simulink model "ardrone_alphaepsilon"  (R2023b)
settings: configuration reference "AR_Drone_ConfigSet" (kept outside this file)
undefined symbols (not defined in the file or in its folder): accelerometerXyzGains, accelerometerXyzOffsets, DiscIntNeverNeededParam, gyroXyzOffsets, Mag_Calib_Gain_Vector, Mag_Calib_Offset_Vector
libraries: simulink x4, AR_Drone_Sensors x2, AR_Drone_Actuators x2, vrlib x2
settings Model: DataDictionary=ArDroneDataDictionary.sldd  EnableAccessToBaseWorkspace=off  SimulationMode=external  ExtModeTrigDuration=48000  Creator=nraman  LastModifiedBy=sonso
settings ConfigSetRef: SourceName=AR_Drone_ConfigSet

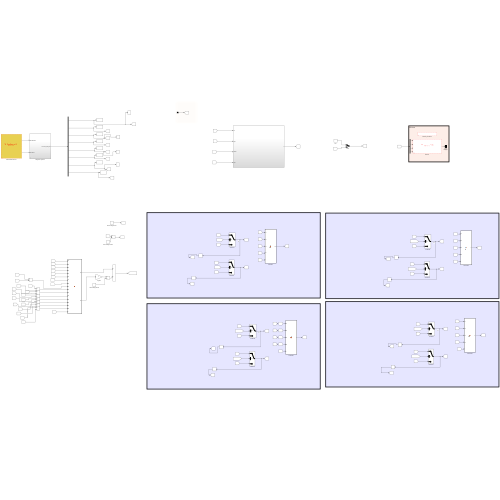
[thumbnail: Simulink's stored preview of the top-level diagram]
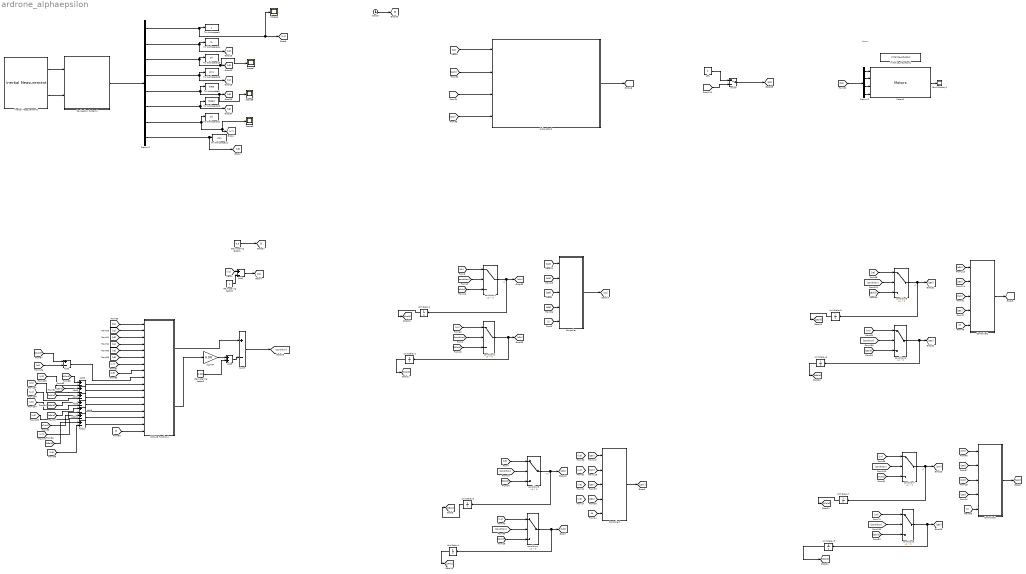
== system ardrone_alphaepsilon ==
  note: Motors
  note: x1
  note: x1
  note: x1
  note: x1
  Add{1..3,6..11} (9 alike) : Sum  Inputs=+-
  Add5 : Sum
  Clock5 : Clock
  Controller : MATLAB Function  TreatAsAtomicUnit=on
  Controller1 : MATLAB Function  TreatAsAtomicUnit=on
  Controller2 : MATLAB Function  TreatAsAtomicUnit=on
  Controller3 : MATLAB Function  TreatAsAtomicUnit=on
  Demux1 : Demux  Outputs=8
  Demux2 : Demux
  Fault Display1 : Display
  Gain-scaling factor1 : Constant  Value=0.5
  Gain-scaling factor2 : Constant
  Gain-scaling factor6 : Constant  Value=0.001
  Inertial Measurement1 : AR_Drone_Sensors/Inertial Measurement  Ts=1/400
  Initialize_Actuators1 : AR_Drone_Actuators/Initialize_Actuators  ShowSpec=on
  MATLAB Function4 : MATLAB Function  TreatAsAtomicUnit=on
  Motors1 : AR_Drone_Actuators/Motors
  Navigation System1 : Subsystem  AncestorBlock=AR_Drone_Positioning/Navigation System
  Scope{6..9} (4 alike) : Scope
  Subsystem2 : Subsystem
  Sum5 : Sum  Inputs=+-
  To Workspace10 : ToWorkspace  VariableName=theta1  SampleTime=-1
  To Workspace11 : ToWorkspace  VariableName=psi  SampleTime=-1
  To Workspace12 : ToWorkspace  VariableName=psi1  SampleTime=-1
  To Workspace14 : ToWorkspace  VariableName=z1  SampleTime=-1
  To Workspace16 : ToWorkspace  VariableName=phi  SampleTime=-1
  To Workspace18 : ToWorkspace  VariableName=phi1  SampleTime=-1
  To Workspace8 : ToWorkspace  VariableName=theta  SampleTime=-1
  To Workspace9 : ToWorkspace  VariableName=z  SampleTime=-1
  Unit Delay{1..8} (8 alike) : UnitDelay  SampleTime=-1  HasFrameUpgradeWarning=on
  condition{1..8} (8 alike) : Switch  Criteria=u2 > Threshold  SaturateOnIntegerOverflow=off  InputSameDT=off
  off1 : Constant  Value=0
  on/off : ManualSwitch
  sigma4 : Gain  Gain=0.08
  wires:
  Inertial Measurement1/1 -> Navigation System1/1(IMU Data Bus)
  Inertial Measurement1/2 -> Navigation System1/2(CheckSum)
  [Uphi] -> Subsystem2/2(Uphi)
  [Utheta] -> Subsystem2/3(Utheta)
  Motors1/1 -> Fault Display1/1
  Demux2/2 -> Motors1/2
  Demux2/3 -> Motors1/3
  Demux2/1 -> Motors1/1
  Demux2/4 -> Motors1/4
  Subsystem2/1(Out1) -> [power]
  [PP] -> Demux2/1
  [Uz] -> Subsystem2/1(Uz)
  Navigation System1/1(Controller_Data_Bus) -> Demux1/1
  Demux1/6 -> [x6], To Workspace10/1
  Demux1/8 -> [x8], To Workspace12/1
  Demux1/4 -> [x4], To Workspace18/1
  Demux1/3 -> [x3], Scope7/1, To Workspace16/1
  Demux1/2 -> [x2], To Workspace14/1
  Demux1/5 -> [x5], Scope8/1, To Workspace8/1
  Demux1/7 -> [x7], Scope9/1, To Workspace11/1
  [r] -> Controller1/5(r)
  [x8] -> condition8/1
  condition7/1 -> Unit Delay7/1, [z7ti]
  [r] -> Controller2/5(r)
  [x5] -> condition5/1
  Unit Delay4/1 -> [z4old]
  Controller3/1(u) -> [Upsi]
  [x1] -> Add1/1
  [z6ti] -> Controller2/2(x2)
  [z7ti] -> Controller3/1(x1)
  condition8/1 -> Unit Delay8/1, [z8ti]
  [z8old] -> condition8/3
  Unit Delay5/1 -> [z5old]
  Unit Delay3/1 -> [z3old]
  [z5ti] -> Controller2/1(x1)
  [z6old] -> condition6/3
  [condition] -> condition8/2
  condition5/1 -> Unit Delay5/1, [z5ti]
  [z8ti] -> Controller3/2(x2)
  condition6/1 -> Unit Delay6/1, [z6ti]
  Controller2/1(u) -> [Utheta]
  Unit Delay6/1 -> [z6old]
  [r] -> Controller3/5(r)
  condition3/1 -> Unit Delay3/1, [z3ti]
  [z7old] -> condition7/3
  Unit Delay7/1 -> [z7old]
  [condition] -> condition7/2
  condition2/1 -> Unit Delay2/1, [z2ti]
  Unit Delay2/1 -> [z2old]
  [condition] -> condition1/2
  [x3] -> condition3/1
  Unit Delay8/1 -> [z8old]
  condition1/1 -> Unit Delay1/1, [z1ti]
  [z4ti] -> Controller1/2(x2)
  [x6] -> condition6/1
  [condition] -> condition3/2
  [z3ti] -> Controller1/1(x1)
  [condition] -> condition6/2
  [r] -> Controller/5(r)
  Add1/1 -> [z1]
  [x7] -> condition7/1
  [z4old] -> condition4/3
  [z2ti] -> Controller/2(x2)
  [z1old] -> condition1/3
  [z1ti] -> Controller/1(x1)
  [z2old] -> condition2/3
  [condition] -> condition2/2
  [condition] -> condition4/2
  [z1] -> condition1/1
  [x4] -> condition4/1
  Gain-scaling factor2/1 -> Add1/2
  Unit Delay1/1 -> [z1old]
  [x2] -> condition2/1
  [z5old] -> condition5/3
  Controller1/1(u) -> [Uphi]
  condition4/1 -> Unit Delay4/1, [z4ti]
  [z3old] -> condition3/3
  [condition] -> condition5/2
  MATLAB Function4/2(Ex) -> sigma4/1
  [r] -> MATLAB Function4/17(r)
  [x8] -> MATLAB Function4/8(x8)
  sigma4/1 -> Add5/1
  Add5/1 -> Sum5/2
  [x7] -> MATLAB Function4/7(x7)
  MATLAB Function4/1(Ee) -> Sum5/1
  Gain-scaling factor6/1 -> Add5/2
  [x5] -> MATLAB Function4/5(x5)
  Add3/1 -> MATLAB Function4/10(e2)
  [z1old] -> Add2/1
  [x6] -> MATLAB Function4/6(x6)
  [z1] -> MATLAB Function4/1(z1)
  [x4] -> MATLAB Function4/4(x4)
  [x3] -> MATLAB Function4/3(x3)
  [x2] -> MATLAB Function4/2(x2)
  [z3ti] -> Controller/3(x3)
  [z5ti] -> Controller/4(x5)
  [z6ti] -> Controller1/3(x6)
  [z8ti] -> Controller1/4(x8)
  [z4ti] -> Controller3/3(x4)
  [z6ti] -> Controller3/4(x6)
  [z4ti] -> Controller2/3(x4)
  [z8ti] -> Controller2/4(x8)
  Sum5/1 -> [condition]
  Gain-scaling factor1/1 -> [r]
  Add2/1 -> MATLAB Function4/9(e1)
  [z1] -> Add2/2
  Add6/1 -> MATLAB Function4/11(e3)
  Add7/1 -> MATLAB Function4/12(e4)
  Add8/1 -> MATLAB Function4/13(e5)
  Add9/1 -> MATLAB Function4/14(e6)
  Add10/1 -> MATLAB Function4/15(e7)
  Add11/1 -> MATLAB Function4/16(e8)
  [x2] -> Add3/2
  [x3] -> Add6/2
  [x4] -> Add7/2
  [x5] -> Add8/2
  [x6] -> Add9/2
  [x7] -> Add10/2
  [x8] -> Add11/2
  [z2old] -> Add3/1
  [z3old] -> Add6/1
  [z4old] -> Add7/1
  [z5old] -> Add8/1
  [z6old] -> Add9/1
  [z7old] -> Add10/1
  [z8old] -> Add11/1
  [power] -> on/off/2
  on/off/1 -> [PP]
  Clock5/1 -> [t]
  off1/1 -> on/off/1
  [Upsi] -> Subsystem2/4(Upsi)
  Demux1/1 -> Scope6/1, [x1], To Workspace9/1
  Controller/1(Uz) -> [Uz]

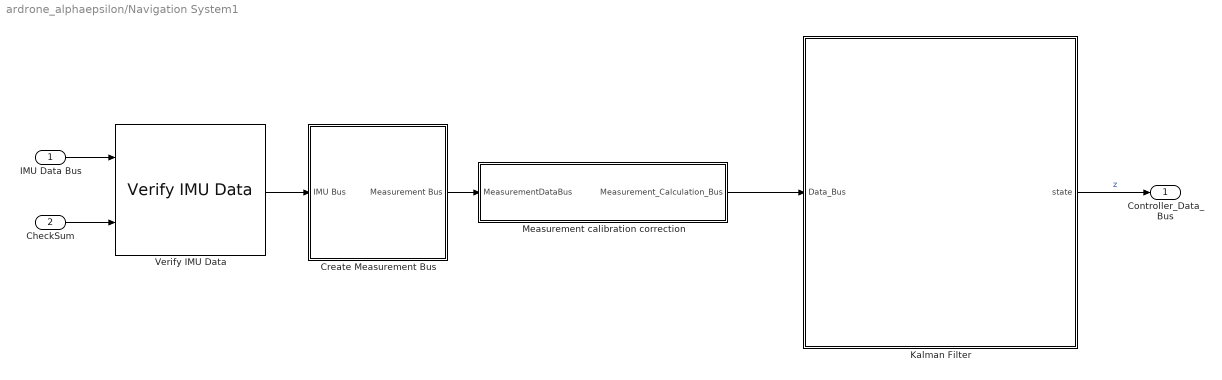
== system ardrone_alphaepsilon/Navigation System1 ==
  IMU Data Bus : Inport  OutDataTypeStr=Bus: IMU_Packets
  CheckSum : Inport  Port=2
  Create Measurement Bus : Subsystem
  Kalman Filter : Subsystem
  Measurement calibration correction : Subsystem
  Verify IMU Data : AR_Drone_Sensors/Verify IMU Data
  Controller_Data_Bus : Outport
  wires:
  Create Measurement Bus/1(Measurement Bus) -> Measurement calibration correction/1(MeasurementDataBus)
  Verify IMU Data/1 -> Create Measurement Bus/1(IMU Bus)
  Kalman Filter/1(state) -> Controller_Data_Bus/1  "z"
  CheckSum/1 -> Verify IMU Data/2
  IMU Data Bus/1 -> Verify IMU Data/1
  Measurement calibration correction/1(Measurement_Calculation_Bus) -> Kalman Filter/1(Data_Bus)

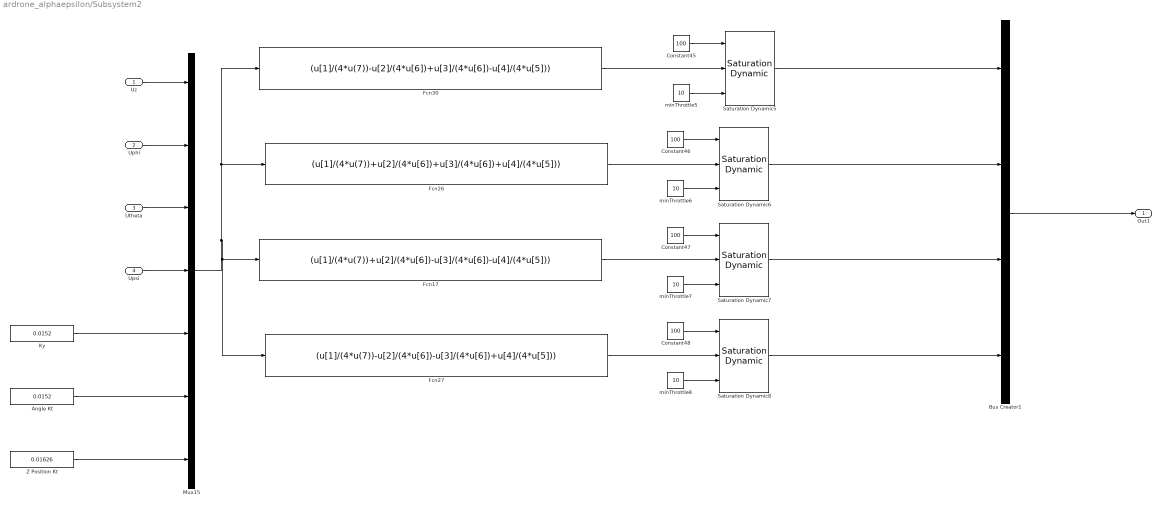
== system ardrone_alphaepsilon/Subsystem2 ==
  Uz : Inport
  Uphi : Inport  Port=2
  Utheta : Inport  Port=3
  Upsi : Inport  Port=4
  Angle Kt : Constant  Value=0.0152
  Bus Creator1 : BusCreator  Inputs=4
  Constant{45..48} (4 alike) : Constant  Value=100  OutDataTypeStr=int16  SampleTime=-1
  Fcn17 : Fcn  Expr=(u[1]/(4*u(7))+u[2]/(4*u[6])-u[3]/(4*u[6])-u[4]/(4*u[5]))
  Fcn26 : Fcn  Expr=(u[1]/(4*u(7))+u[2]/(4*u[6])+u[3]/(4*u[6])+u[4]/(4*u[5]))
  Fcn27 : Fcn  Expr=(u[1]/(4*u(7))-u[2]/(4*u[6])-u[3]/(4*u[6])+u[4]/(4*u[5]))
  Fcn30 : Fcn  Expr=(u[1]/(4*u(7))-u[2]/(4*u[6])+u[3]/(4*u[6])-u[4]/(4*u[5]))
  Ky : Constant  Value=0.0152
  Mux15 : Mux  Inputs=7
  Saturation Dynamic{5..8} (4 alike) : simulink/Discontinuities/Saturation Dynamic  OutMin=[]  OutMax=[]  OutDataTypeStr=Inherit: Same as second input  OutDataType=fixdt(1, 16)  OutScaling=2^-10  DoSatur=off
  Z Position Kt : Constant  Value=0.01626
  minThrottle{5..8} (4 alike) : Constant  Value=10  OutDataTypeStr=int16
  Out1 : Outport
  wires:
  Fcn27/1 -> Saturation Dynamic8/2
  Constant47/1 -> Saturation Dynamic7/1
  Constant45/1 -> Saturation Dynamic5/1
  minThrottle7/1 -> Saturation Dynamic7/3
  Constant48/1 -> Saturation Dynamic8/1
  Fcn26/1 -> Saturation Dynamic6/2
  minThrottle8/1 -> Saturation Dynamic8/3
  Mux15/1 -> Fcn17/1, Fcn27/1, Fcn30/1, Fcn26/1
  minThrottle6/1 -> Saturation Dynamic6/3
  minThrottle5/1 -> Saturation Dynamic5/3
  Fcn30/1 -> Saturation Dynamic5/2
  Constant46/1 -> Saturation Dynamic6/1
  Fcn17/1 -> Saturation Dynamic7/2
  Saturation Dynamic6/1 -> Bus Creator1/2
  Bus Creator1/1 -> Out1/1
  Ky/1 -> Mux15/5
  Saturation Dynamic5/1 -> Bus Creator1/1
  Saturation Dynamic7/1 -> Bus Creator1/3
  Angle Kt/1 -> Mux15/6
  Saturation Dynamic8/1 -> Bus Creator1/4
  ? -> ?
  Uz/1 -> Mux15/1
  Z Position Kt/1 -> Mux15/7
  Uphi/1 -> Mux15/2
  Utheta/1 -> Mux15/3
  Upsi/1 -> Mux15/4

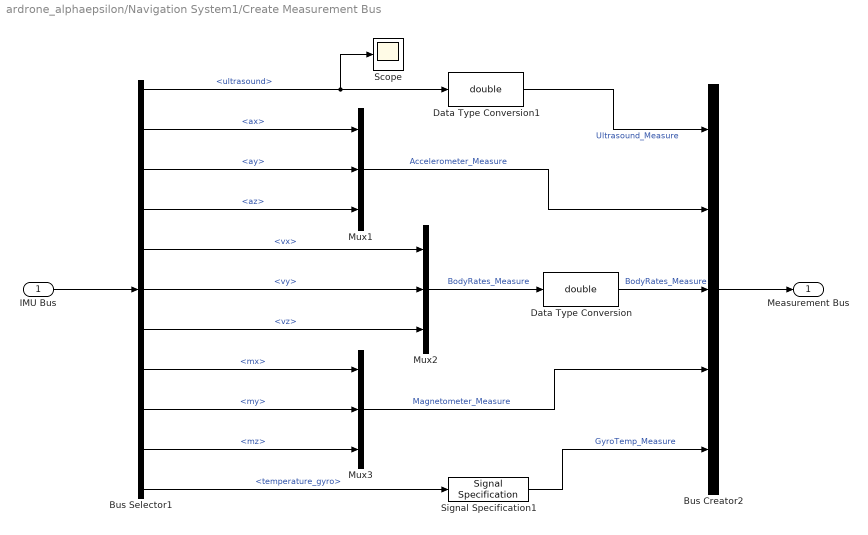
== system ardrone_alphaepsilon/Navigation System1/Create Measurement Bus ==
  IMU Bus : Inport
  Bus Creator2 : BusCreator  Inputs=5
  Bus Selector1 : BusSelector  OutputSignals=ultrasound,ax,ay,az,vx,vy,vz,mx,my,mz,temperature_gyro
  Data Type Conversion : DataTypeConversion  OutDataTypeStr=double  SaturateOnIntegerOverflow=off  RndMeth=Floor
  Data Type Conversion1 : DataTypeConversion  OutDataTypeStr=double  SaturateOnIntegerOverflow=off  RndMeth=Floor
  Mux1 : Mux  Inputs=3
  Mux2 : Mux  Inputs=3
  Mux3 : Mux  Inputs=3
  Scope : Scope
  Signal Specification1 : SignalSpecification
  Measurement Bus : Outport
  wires:
  Mux1/1 -> Bus Creator2/2  "Accelerometer_Measure"
  Bus Selector1/2 -> Mux1/1  "<ax>"
  Mux3/1 -> Bus Creator2/4  "Magnetometer_Measure"
  Data Type Conversion/1 -> Bus Creator2/3  "BodyRates_Measure"
  Bus Selector1/3 -> Mux1/2  "<ay>"
  Signal Specification1/1 -> Bus Creator2/5  "GyroTemp_Measure"
  Bus Selector1/4 -> Mux1/3  "<az>"
  Bus Selector1/9 -> Mux3/2  "<my>"
  Bus Selector1/10 -> Mux3/3  "<mz>"
  Bus Selector1/8 -> Mux3/1  "<mx>"
  IMU Bus/1 -> Bus Selector1/1
  Bus Selector1/5 -> Mux2/1  "<vx>"
  Bus Selector1/7 -> Mux2/3  "<vz>"
  Bus Selector1/6 -> Mux2/2  "<vy>"
  Bus Selector1/1 -> Scope/1, Data Type Conversion1/1  "<ultrasound>"
  Bus Selector1/11 -> Signal Specification1/1  "<temperature_gyro>"
  Data Type Conversion1/1 -> Bus Creator2/1  "Ultrasound_Measure"
  Bus Creator2/1 -> Measurement Bus/1
  Mux2/1 -> Data Type Conversion/1  "BodyRates_Measure"

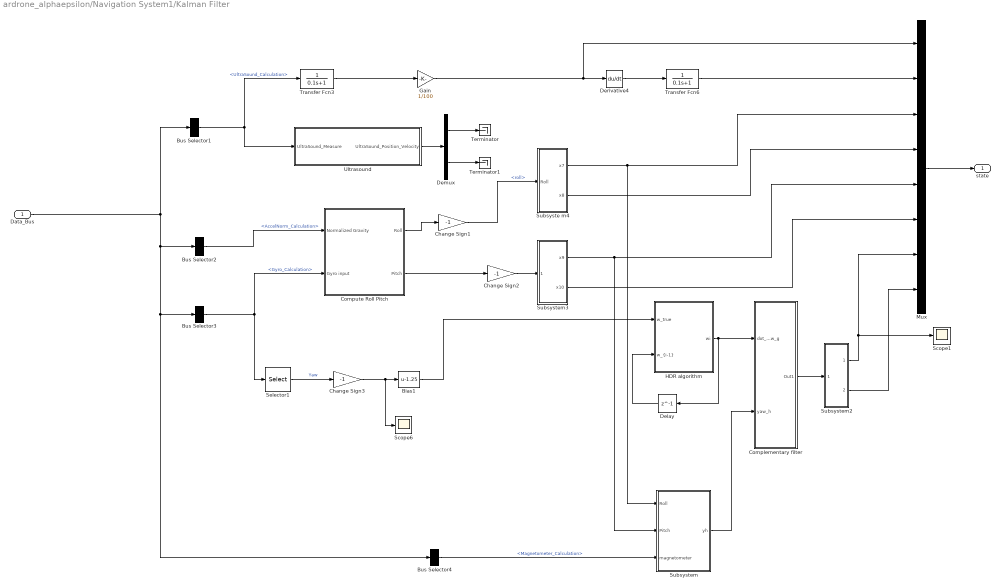
== system ardrone_alphaepsilon/Navigation System1/Kalman Filter ==
  Data_Bus : Inport
  Bias1 : Bias  Bias=-1.25  SaturateOnIntegerOverflow=off
  Bus Selector1 : BusSelector  OutputSignals=UltraSound_Calculation
  Bus Selector2 : BusSelector  OutputSignals=AccelNorm_Calculation
  Bus Selector3 : BusSelector  OutputSignals=Gyro_Calculation
  Bus Selector4 : BusSelector  OutputSignals=Magnetometer_Calculation
  Change Sign1 : Gain  Gain=-1
  Change Sign2 : Gain  Gain=-1
  Change Sign3 : Gain  Gain=-1
  Complementary filter : Subsystem
  Compute Roll Pitch : Subsystem
  Delay : Delay  DelayLength=1  InitialCondition=0
  Demux : Demux  Outputs=2
  Derivative4 : Derivative
  Gain : Gain  Gain=1/100
  HDR algorithm : Subsystem
  Mux : Mux  Inputs=8
  Scope1 : Scope
  Scope6 : Scope
  Selector1 : Selector  IndexMode=Zero-based  InputPortWidth=3  IndexOptions=Index vector (dialog)  Indices=[2]  OutputSizes=1
  Subsyste m4 : Subsystem
  Subsystem : Subsystem
  Subsystem2 : Subsystem
  Subsystem3 : Subsystem
  Terminator : Terminator
  Terminator1 : Terminator
  Transfer Fcn3 : TransferFcn  Denominator=[0.1 1]
  Transfer Fcn6 : TransferFcn  Denominator=[0.1 1]
  "Ultrasound  " : Subsystem
  state : Outport
  wires:
  Compute Roll Pitch/2(Pitch) -> Change Sign2/1
  Compute Roll Pitch/1(Roll) -> Change Sign1/1
  Demux/1 -> Terminator/1
  Demux/2 -> Terminator1/1
  "Ultrasound  "/1("UltraSound_Position_Velocity ") -> Demux/1
  Bus Selector2/1 -> Compute Roll Pitch/1(Normalized Gravity)  "<AccelNorm_Calculation>"
  Selector1/1 -> Change Sign3/1  "Yaw"
  Bus Selector3/1 -> Selector1/1, Compute Roll Pitch/2(Gyro input)  "<Gyro_Calculation>"
  Data_Bus/1 -> Bus Selector1/1, Bus Selector2/1, Bus Selector4/1, Bus Selector3/1
  Bias1/1 -> HDR algorithm/1(w_true)
  Complementary filter/1(Out1) -> Subsystem2/1(yaw)
  Subsystem/1(yh) -> Complementary filter/2(yaw_h)
  Change Sign3/1 -> Scope6/1, Bias1/1
  Bus Selector4/1 -> Subsystem/3(magnetometer)  "<Magnetometer_Calculation>"
  Delay/1 -> HDR algorithm/2("w_{i-1}")
  HDR algorithm/1(wi) -> Delay/1, Complementary filter/1(dot_Yaw_g)
  Bus Selector1/1 -> "Ultrasound  "/1(UltraSound_Measure), Transfer Fcn3/1  "<UltraSound_Calculation>"
  Gain/1 -> Mux/1, Derivative4/1
  Derivative4/1 -> Transfer Fcn6/1
  Transfer Fcn3/1 -> Gain/1
  Transfer Fcn6/1 -> Mux/2
  Subsystem3/2(x10) -> Mux/6
  Subsystem3/1(x9) -> Mux/5, Subsystem/2(Pitch)
  Subsyste m4/1(x7) -> Mux/3, Subsystem/1(Roll)
  Change Sign1/1 -> Subsyste m4/1("Roll ")  "<roll>"
  Change Sign2/1 -> Subsystem3/1(Pitch)
  Mux/1 -> state/1
  Subsyste m4/2(x8) -> Mux/4
  Subsystem2/2(x12) -> Mux/8
  Subsystem2/1(x11) -> Mux/7, Scope1/1

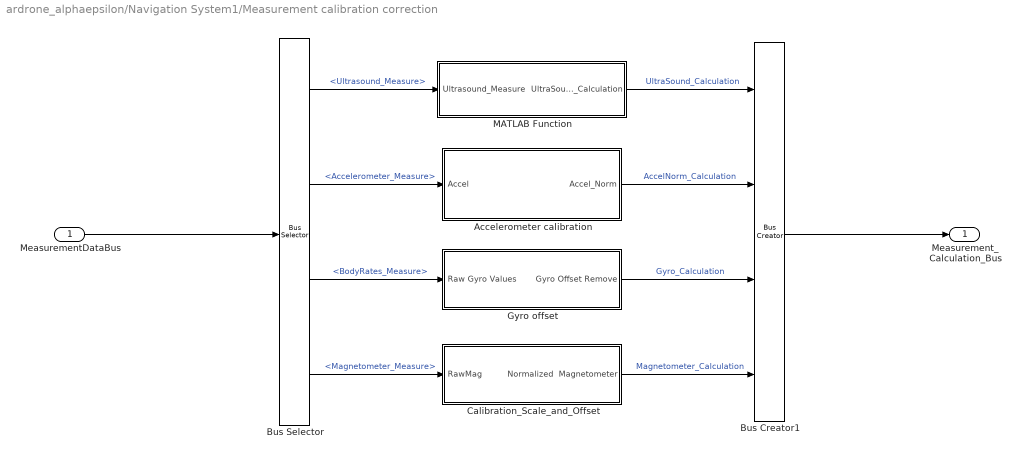
== system ardrone_alphaepsilon/Navigation System1/Measurement calibration correction ==
  MeasurementDataBus : Inport
  Accelerometer calibration : Subsystem
  Bus Creator1 : BusCreator  Inputs=4
  Bus Selector : BusSelector  OutputSignals=Ultrasound_Measure,Accelerometer_Measure,BodyRates_Measure,Magnetometer_Measure
  Calibration_Scale_and_Offset : Subsystem
  Gyro offset : Subsystem
  MATLAB Function : MATLAB Function  TreatAsAtomicUnit=on
  Measurement_Calculation_Bus : Outport
  wires:
  Bus Selector/1 -> MATLAB Function/1(Ultrasound_Measure)  "<Ultrasound_Measure>"
  Gyro offset/1(Gyro Offset Remove) -> Bus Creator1/3  "Gyro_Calculation"
  Bus Selector/2 -> Accelerometer calibration/1(Accel)  "<Accelerometer_Measure>"
  Accelerometer calibration/1(Accel_Norm) -> Bus Creator1/2  "AccelNorm_Calculation"
  MATLAB Function/1(UltraSound_Calculation) -> Bus Creator1/1  "UltraSound_Calculation"
  Calibration_Scale_and_Offset/1(Normalized  Magnetometer) -> Bus Creator1/4  "Magnetometer_Calculation"
  MeasurementDataBus/1 -> Bus Selector/1
  Bus Selector/3 -> Gyro offset/1(Raw Gyro Values)  "<BodyRates_Measure>"
  Bus Creator1/1 -> Measurement_Calculation_Bus/1
  Bus Selector/4 -> Calibration_Scale_and_Offset/1(RawMag)  "<Magnetometer_Measure>"

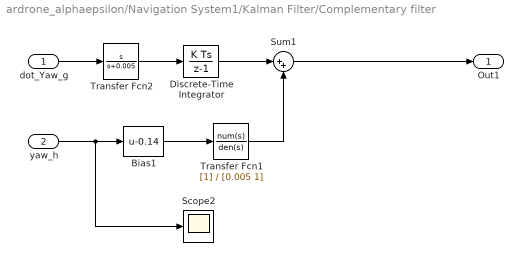
== system ardrone_alphaepsilon/Navigation System1/Kalman Filter/Complementary filter ==
  dot_Yaw_g : Inport
  yaw_h : Inport  Port=2
  Bias1 : Bias  Bias=-0.14  SaturateOnIntegerOverflow=off
  Discrete-Time Integrator : DiscreteIntegrator  SampleTime=0.0025  ICPrevOutput=DiscIntNeverNeededParam  ICPrevScaledInput=DiscIntNeverNeededParam
  Scope2 : Scope
  Sum1 : Sum  Inputs=|++
  Transfer Fcn1 : TransferFcn  Denominator=[0.005 1]
  Transfer Fcn2 : TransferFcn  Numerator=[1 0]  Denominator=[1 0.005]
  Out1 : Outport
  wires:
  yaw_h/1 -> Bias1/1, Scope2/1
  dot_Yaw_g/1 -> Transfer Fcn2/1
  Discrete-Time Integrator/1 -> Sum1/1
  Transfer Fcn2/1 -> Discrete-Time Integrator/1
  Transfer Fcn1/1 -> Sum1/2
  Bias1/1 -> Transfer Fcn1/1
  Sum1/1 -> Out1/1

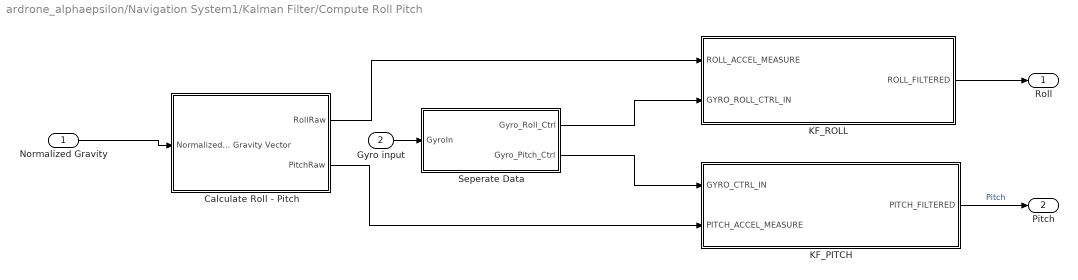
== system ardrone_alphaepsilon/Navigation System1/Kalman Filter/Compute Roll Pitch ==
  Normalized Gravity : Inport
  Gyro input : Inport  Port=2
  Calculate Roll - Pitch : Subsystem
  KF_PITCH : Subsystem
  KF_ROLL : Subsystem
  Seperate Data : Subsystem
  Roll : Outport
  Pitch : Outport  Port=2
  wires:
  Seperate Data/2(Gyro_Pitch_Ctrl) -> KF_PITCH/1(GYRO_CTRL_IN)
  Calculate Roll - Pitch/1(RollRaw) -> KF_ROLL/1(ROLL_ACCEL_MEASURE)
  Calculate Roll - Pitch/2(PitchRaw) -> KF_PITCH/2(PITCH_ACCEL_MEASURE)
  Gyro input/1 -> Seperate Data/1(GyroIn)
  Normalized Gravity/1 -> Calculate Roll - Pitch/1(Normalized Gravity Vector)
  KF_ROLL/1(ROLL_FILTERED) -> Roll/1
  KF_PITCH/1(PITCH_FILTERED) -> Pitch/1  "Pitch"
  Seperate Data/1(Gyro_Roll_Ctrl) -> KF_ROLL/2(GYRO_ROLL_CTRL_IN)

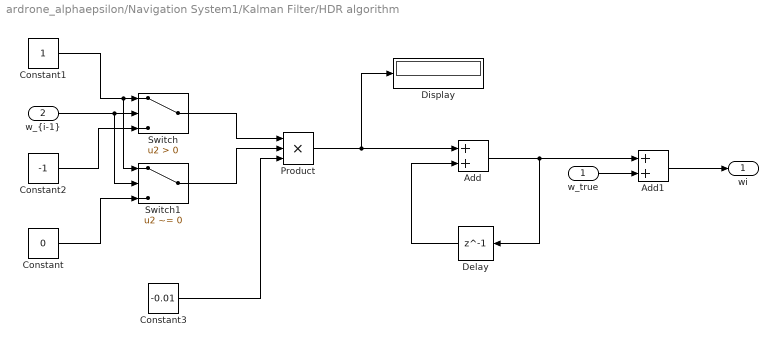
== system ardrone_alphaepsilon/Navigation System1/Kalman Filter/HDR algorithm ==
  w_true : Inport
  "w_{i-1}" : Inport  Port=2
  Add : Sum
  Add1 : Sum
  Constant : Constant  Value=0
  Constant1 : Constant
  Constant2 : Constant  Value=-1
  Constant3 : Constant  Value=-0.01
  Delay : Delay  DelayLength=1  InitialCondition=0
  Display : Display
  Product : Product  Inputs=3
  Switch : Switch  Criteria=u2 > Threshold  SaturateOnIntegerOverflow=off  InputSameDT=off
  Switch1 : Switch  Criteria=u2 ~= 0  SaturateOnIntegerOverflow=off  InputSameDT=off
  wi : Outport
  wires:
  "w_{i-1}"/1 -> Switch1/2, Switch/2
  Constant1/1 -> Switch1/1, Switch/1
  Constant2/1 -> Switch/3
  Switch/1 -> Product/1
  Switch1/1 -> Product/2
  Constant/1 -> Switch1/3
  Constant3/1 -> Product/3
  Add/1 -> Add1/1, Delay/1
  Delay/1 -> Add/2
  w_true/1 -> Add1/2
  Add1/1 -> wi/1
  Product/1 -> Display/1, Add/1

== system ardrone_alphaepsilon/Navigation System1/Kalman Filter/Subsyste m4 ==
  "Roll " : Inport
  Derivative13 : Derivative
  Gain2 : Gain  Gain=pi/180
  Roll : Scope
  Transfer Fcn1 : TransferFcn  Numerator=[0.5]  Denominator=[0.25 1]
  x7 : Outport
  x8 : Outport  Port=2
  wires:
  Transfer Fcn1/1 -> x8/1
  Derivative13/1 -> Transfer Fcn1/1
  "Roll "/1 -> Gain2/1, Roll/1
  Gain2/1 -> x7/1, Derivative13/1

== system ardrone_alphaepsilon/Navigation System1/Kalman Filter/Subsystem ==
  Roll : Inport
  Pitch : Inport  Port=2
  magnetometer : Inport  Port=3
  Demux : Demux  Outputs=3
  Fcn : Fcn  Expr=atan((-u(4)*cos(u(1))+u(5)*sin(u(1)))/(u(3)*cos(u(2))+u(4)*sin(u(1))*sin(u(2))+u(5)*sin(u(2))*cos(u(1))))
  Mux : Mux  Inputs=5
  yh : Outport
  wires:
  magnetometer/1 -> Demux/1
  Demux/3 -> Mux/5
  Demux/2 -> Mux/4
  Demux/1 -> Mux/3
  Pitch/1 -> Mux/2
  Roll/1 -> Mux/1
  Mux/1 -> Fcn/1
  Fcn/1 -> yh/1

== system ardrone_alphaepsilon/Navigation System1/Kalman Filter/Subsystem2 ==
  yaw : Inport
  Derivative1 : Derivative
  Gain3 : Gain  Gain=pi/180
  Transfer Fcn5 : TransferFcn  Denominator=[0.1 1]
  x11 : Outport
  x12 : Outport  Port=2
  wires:
  yaw/1 -> Gain3/1
  Gain3/1 -> x11/1, Derivative1/1
  Derivative1/1 -> Transfer Fcn5/1
  Transfer Fcn5/1 -> x12/1

== system ardrone_alphaepsilon/Navigation System1/Kalman Filter/Subsystem3 ==
  Pitch : Inport
  Derivative13 : Derivative
  Gain2 : Gain  Gain=pi/180
  Pitch1 : Scope
  Transfer Fcn1 : TransferFcn  Numerator=[0.5]  Denominator=[0.25 1]
  x9 : Outport
  x10 : Outport  Port=2
  wires:
  Pitch/1 -> Gain2/1, Pitch1/1
  Derivative13/1 -> Transfer Fcn1/1
  Transfer Fcn1/1 -> x10/1
  Gain2/1 -> x9/1, Derivative13/1

== system ardrone_alphaepsilon/Navigation System1/Kalman Filter/Ultrasound   ==
  UltraSound_Measure : Inport
  Kalman Tracker : MATLAB Function  TreatAsAtomicUnit=on
  Unit Delay1 : UnitDelay  InitialCondition=[0 0 ]  SampleTime=-1  HasFrameUpgradeWarning=on
  Unit Delay2 : UnitDelay  InitialCondition=eye(2)  SampleTime=-1  HasFrameUpgradeWarning=on
  "UltraSound_Position_Velocity " : Outport
  wires:
  Unit Delay1/1 -> Kalman Tracker/3(state_correction_input), "UltraSound_Position_Velocity "/1
  Unit Delay2/1 -> Kalman Tracker/2(covariance_correction_input)
  UltraSound_Measure/1 -> Kalman Tracker/1(UltraSoundMeasure)
  Kalman Tracker/1(state_correction) -> Unit Delay1/1
  Kalman Tracker/2(covariance_correction) -> Unit Delay2/1

== system ardrone_alphaepsilon/Navigation System1/Measurement calibration correction/Accelerometer calibration ==
  Accel : Inport
  Apply calibration parameters : Subsystem
  Data Type Conversion : DataTypeConversion  OutDataTypeStr=double  SaturateOnIntegerOverflow=off  RndMeth=Floor
  Low pass filter : Subsystem
  Normalize Vector : vrlib/Utilities/Normalize Vector  maxzero=0
  Accel_Norm : Outport
  wires:
  Accel/1 -> Data Type Conversion/1
  Data Type Conversion/1 -> Apply calibration parameters/1(Raw Accelerometer Data)
  Apply calibration parameters/1(Calibrated Accelerometer Data) -> Low pass filter/1(Offset Accel)
  Low pass filter/1(Filtered Accel) -> Normalize Vector/1
  Normalize Vector/1 -> Accel_Norm/1

== system ardrone_alphaepsilon/Navigation System1/Measurement calibration correction/Calibration_Scale_and_Offset ==
  RawMag : Inport
  Normalize Vector : vrlib/Utilities/Normalize Vector  maxzero=0
  Process Magnetometer : Subsystem
  Normalized  Magnetometer : Outport
  wires:
  RawMag/1 -> Process Magnetometer/1(Magnetometer)
  Process Magnetometer/1(MagVector) -> Normalize Vector/1
  Normalize Vector/1 -> Normalized  Magnetometer/1

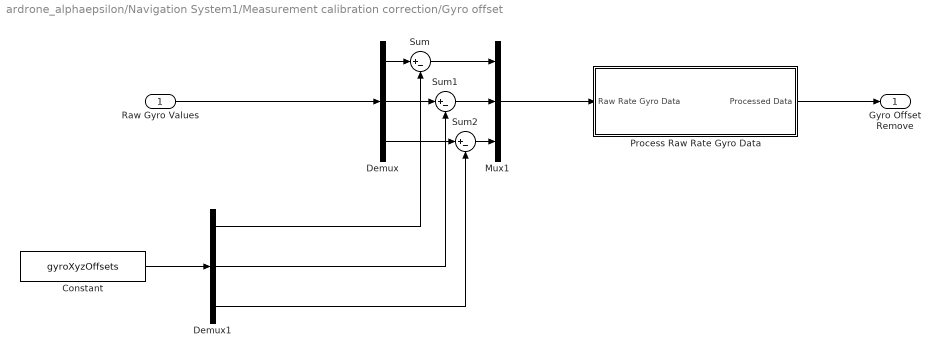
== system ardrone_alphaepsilon/Navigation System1/Measurement calibration correction/Gyro offset ==
  Raw Gyro Values : Inport
  Constant : Constant  Value=gyroXyzOffsets  VectorParams1D=off
  Demux : Demux  Outputs=3
  Demux1 : Demux  Outputs=3
  Mux1 : Mux  Inputs=3
  Process Raw Rate Gyro Data : Subsystem
  Sum : Sum  Inputs=|+-
  Sum1 : Sum  Inputs=|+-
  Sum2 : Sum  Inputs=|+-
  Gyro Offset Remove : Outport
  wires:
  Demux/3 -> Sum2/1
  Sum1/1 -> Mux1/2
  Demux1/1 -> Sum/2
  Sum2/1 -> Mux1/3
  Demux/2 -> Sum1/1
  Demux/1 -> Sum/1
  Sum/1 -> Mux1/1
  Mux1/1 -> Process Raw Rate Gyro Data/1(Raw Rate Gyro Data)
  Demux1/2 -> Sum1/2
  Demux1/3 -> Sum2/2
  Process Raw Rate Gyro Data/1(Processed Data) -> Gyro Offset Remove/1
  Constant/1 -> Demux1/1
  Raw Gyro Values/1 -> Demux/1

== system ardrone_alphaepsilon/Navigation System1/Kalman Filter/Compute Roll Pitch/Calculate Roll - Pitch ==
  note: http://www.digikey.com/en/articles/techzone/2011/may/using-an-accelerometer-for-inclination-sensing
  Normalized Gravity Vector : Inport
  Gain4 : Gain  Gain=180/pi
  Gain5 : Gain  Gain=-180/pi
  MATLAB Function : MATLAB Function  TreatAsAtomicUnit=on
  RollRaw : Outport
  PitchRaw : Outport  Port=2
  wires:
  Gain5/1 -> PitchRaw/1
  Gain4/1 -> RollRaw/1
  MATLAB Function/2(Pitch) -> Gain5/1  "roll"
  MATLAB Function/1(Roll) -> Gain4/1  "pitch"
  Normalized Gravity Vector/1 -> MATLAB Function/1(Ax_Ay_Az)

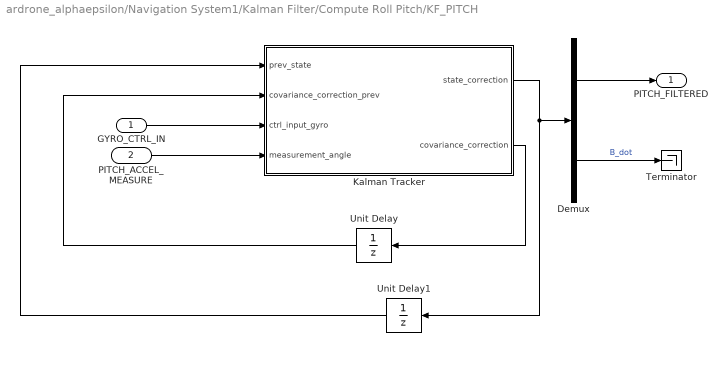
== system ardrone_alphaepsilon/Navigation System1/Kalman Filter/Compute Roll Pitch/KF_PITCH ==
  GYRO_CTRL_IN : Inport
  PITCH_ACCEL_MEASURE : Inport  Port=2
  Demux : Demux  Outputs=2
  Kalman Tracker : MATLAB Function  TreatAsAtomicUnit=on
  Terminator : Terminator
  Unit Delay : UnitDelay  InitialCondition=eye(2)  SampleTime=-1  HasFrameUpgradeWarning=on
  Unit Delay1 : UnitDelay  InitialCondition=[0 0]'  SampleTime=-1  HasFrameUpgradeWarning=on
  PITCH_FILTERED : Outport
  wires:
  Demux/2 -> Terminator/1  "B_dot"
  PITCH_ACCEL_MEASURE/1 -> Kalman Tracker/4(measurement_angle)
  Unit Delay/1 -> Kalman Tracker/2(covariance_correction_prev)
  GYRO_CTRL_IN/1 -> Kalman Tracker/3(ctrl_input_gyro)
  Unit Delay1/1 -> Kalman Tracker/1(prev_state)
  Kalman Tracker/1(state_correction) -> Demux/1, Unit Delay1/1
  Demux/1 -> PITCH_FILTERED/1
  Kalman Tracker/2(covariance_correction) -> Unit Delay/1

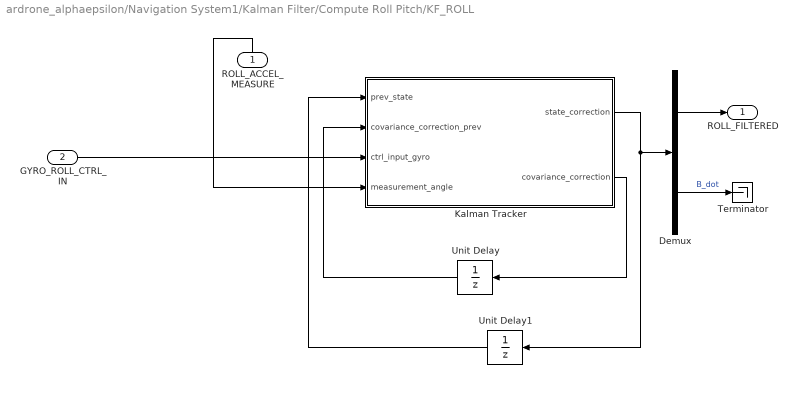
== system ardrone_alphaepsilon/Navigation System1/Kalman Filter/Compute Roll Pitch/KF_ROLL ==
  ROLL_ACCEL_MEASURE : Inport
  GYRO_ROLL_CTRL_IN : Inport  Port=2
  Demux : Demux  Outputs=2
  Kalman Tracker : MATLAB Function  TreatAsAtomicUnit=on
  Terminator : Terminator
  Unit Delay : UnitDelay  InitialCondition=eye(2)  SampleTime=-1  HasFrameUpgradeWarning=on
  Unit Delay1 : UnitDelay  InitialCondition=[0 0]'  SampleTime=-1  HasFrameUpgradeWarning=on
  ROLL_FILTERED : Outport
  wires:
  Demux/2 -> Terminator/1  "B_dot"
  Demux/1 -> ROLL_FILTERED/1
  ROLL_ACCEL_MEASURE/1 -> Kalman Tracker/4(measurement_angle)
  Unit Delay/1 -> Kalman Tracker/2(covariance_correction_prev)
  GYRO_ROLL_CTRL_IN/1 -> Kalman Tracker/3(ctrl_input_gyro)
  Unit Delay1/1 -> Kalman Tracker/1(prev_state)
  Kalman Tracker/1(state_correction) -> Demux/1, Unit Delay1/1
  Kalman Tracker/2(covariance_correction) -> Unit Delay/1

== system ardrone_alphaepsilon/Navigation System1/Kalman Filter/Compute Roll Pitch/Seperate Data ==
  GyroIn : Inport
  Demux1 : Demux  Outputs=[1 1]
  Selector2 : Selector  IndexMode=Zero-based  InputPortWidth=3  IndexOptions=Index vector (dialog)  Indices=[0 1]  OutputSizes=1
  Gyro_Roll_Ctrl : Outport
  Gyro_Pitch_Ctrl : Outport  Port=2
  wires:
  Selector2/1 -> Demux1/1
  Demux1/2 -> Gyro_Pitch_Ctrl/1  "GYRO_Y"
  Demux1/1 -> Gyro_Roll_Ctrl/1  "GYRO_X"
  GyroIn/1 -> Selector2/1

== system ardrone_alphaepsilon/Navigation System1/Measurement calibration correction/Accelerometer calibration/Apply calibration parameters ==
  Raw Accelerometer Data : Inport
  Acclerometer Calibration Gains : Constant  Value=accelerometerXyzGains
  Acclerometer Calibration Offsets : Constant  Value=accelerometerXyzOffsets
  Add : Sum  Inputs=+-
  Divide : Product  Inputs=*/
  Invert Axes Definition : Gain  Gain=-1
  Calibrated Accelerometer Data : Outport
  wires:
  Invert Axes Definition/1 -> Calibrated Accelerometer Data/1
  Raw Accelerometer Data/1 -> Add/1
  Acclerometer Calibration Gains/1 -> Divide/2
  Acclerometer Calibration Offsets/1 -> Add/2
  Divide/1 -> Invert Axes Definition/1
  Add/1 -> Divide/1

== system ardrone_alphaepsilon/Navigation System1/Measurement calibration correction/Accelerometer calibration/Low pass filter ==
  Offset Accel : Inport
  Add : Sum
  Gain : Gain  Gain=0.8
  Gain1 : Gain  Gain=0.2
  Unit Delay : UnitDelay  SampleTime=-1  HasFrameUpgradeWarning=on
  Filtered Accel : Outport
  wires:
  Unit Delay/1 -> Gain/1
  Add/1 -> Unit Delay/1, Filtered Accel/1
  Gain1/1 -> Add/1
  Gain/1 -> Add/2
  Offset Accel/1 -> Gain1/1

== system ardrone_alphaepsilon/Navigation System1/Measurement calibration correction/Calibration_Scale_and_Offset/Process Magnetometer ==
  note: magnetometer[ 0 ] = - ( float ) navdata.mx ;
      | magnetometer[ 1 ] = ( float ) navdata.my ;
      | magnetometer[ 2 ] = - ( float ) navdata.mz ;
      | const float Sensitivity[ 3 ] = { 0.0071492608 , 0.0070882491 , 0.0074057781 } ;
      | const float Neutral[ 3 ] = { 118.0 , - 65.0 , 110.0 } ;
  Magnetometer : Inport
  Constant : Constant  Value=[Mag_Calib_Offset_Vector.Gain_X Mag_Calib_Offset_Vector.Gain_Y Mag_Calib_Offset_Vector.Gain_Z]
      settings: AttributesFormatString=%<Value>
  Constant1 : Constant  Value=[Mag_Calib_Gain_Vector.Gain_X Mag_Calib_Gain_Vector.Gain_Y Mag_Calib_Gain_Vector.Gain_Z]
      settings: AttributesFormatString=%<Value>
  Divide : Product  Inputs=/*
  Sum : Sum  Inputs=|+-
  MagVector : Outport
  wires:
  Divide/1 -> MagVector/1
  Constant1/1 -> Divide/1
  Constant/1 -> Sum/2
  Magnetometer/1 -> Sum/1
  Sum/1 -> Divide/2

== system ardrone_alphaepsilon/Navigation System1/Measurement calibration correction/Gyro offset/Process Raw Rate Gyro Data ==
  note: const float Sensitivity[ 3 ] = { 0.0609 , 0.0609 , 0.0609 } ;
  Raw Rate Gyro Data : Inport
  Gain : Gain  Gain=[0.0609, 0.0609, 0.0609]  ParamDataTypeStr=double
  Processed Data : Outport
  wires:
  Raw Rate Gyro Data/1 -> Gain/1
  Gain/1 -> Processed Data/1

== matlab function ardrone_alphaepsilon/Controller3 ==
  data: x1 input; u output; x2 input; x4 input; x6 input; r input
function u  = fcn(x1,x2,x4,x6,r)
Ix =0.0022;
Iy=0.003;
Iz=0.0048;
L=0.1785;
k1=-0;
k2=-0;

upsi=(k1*(x1))/(r^2)+(k2*x2)/(r^1) ;

u=(upsi*Iz-x4*x6*(Ix-Iy));

== matlab function ardrone_alphaepsilon/MATLAB Function4 ==
  data: z1 input; x2 input; x3 input; x4 input; x5 input; x6 input; x7 input; x8 input; e1 input; e2 input; e3 input; e4 input; e5 input; e6 input; e7 input; e8 input; r input; Ee output; Ex output
function [Ee,Ex]   = fcn(z1,x2,x3,x4,x5,x6,x7,x8,e1,e2,e3,e4,e5,e6,e7,e8,r)



Ee=sqrt(e1^2+(e2*r)^2+e3^2+(e4*r)^2+e5^2+(e6*r)^2+e7^2+(e8*r)^2);

Ex=sqrt(z1^2+(x2*r)^2+(x3)^2+(x4*r)^2+(x5)^2+(x6*r)^2+(x7)^2+(x8*r)^2);

== matlab function ardrone_alphaepsilon/Controller ==
  data: x1 input; Uz output; x2 input; x3 input; x5 input; r input
function Uz  = fcn(x1,x2,x3,x5,r)

k1=-84;
k2=-64;

uz=(k1*(x1))/(r^2)+(k2*x2)/(r^1) ;
Uz=((uz+9.81)*0.4290)/(cos(x3)*cos(x5));

== matlab function ardrone_alphaepsilon/Controller1 ==
  data: x1 input; u output; x2 input; x6 input; x8 input; r input
function u  = fcn(x1,x2,x6,x8,r)
Ix =0.0022;
Iy=0.003;
Iz=0.0048;
L=0.1785;
k1=-70;
k2=-25;

uphi=(k1*x1)/(r^2)+(k2*x2)/(r^1) ;
u=(uphi*Ix-x6*x8*(Iy-Iz))/L;

== matlab function ardrone_alphaepsilon/Controller2 ==
  data: x1 input; u output; x2 input; x4 input; x8 input; r input
function u  = fcn(x1,x2,x4,x8,r)
Ix =0.0022;
Iy=0.003;
Iz=0.0048;
L=0.1785;
k1=-50;
k2=-20;

utheta=(k1*(x1))/(r^2)+(k2*x2)/(r^1) ;
u=(utheta*Iy-x4*x8*(Iz-Ix))/L;

== matlab function ardrone_alphaepsilon/Navigation System1/Kalman Filter/Compute Roll Pitch/Calculate Roll - Pitch/MATLAB Function ==
  data: Ax_Ay_Az input; Roll output; Pitch output
function [Roll,Pitch] = CalculateAngle(Ax_Ay_Az)
%#codegen
Ax = -Ax_Ay_Az(1);
Ay = -Ax_Ay_Az(2);
Az = Ax_Ay_Az(3);

Pitch = atan( Ax / sqrt( Ay^2 + Az^2));
Roll = atan( Ay / sqrt( Ax^2 + Az^2));

== matlab function ardrone_alphaepsilon/Navigation System1/Kalman Filter/Compute Roll Pitch/KF_PITCH/Kalman Tracker ==
  data: prev_state input; covariance_correction_prev input; state_correction output; covariance_correction output; ctrl_input_gyro input; measurement_angle input
function [state_correction, covariance_correction] = fcn(prev_state, covariance_correction_prev, ctrl_input_gyro, measurement_angle)


%-------------------------------
%-------------------------------
%---- Predict Stage ------------
%-------------------------------
%-------------------------------
% pix_value = 5;
Ts = 1/400;
%Process Noise
p_var =0.01;
Q = [p_var^2     0         
      0         p_var^2];

%A matrix
A =  [1   -Ts 
      0   1];

%odutput these values with a unit delay (for algebraic loop), apply initial conditions
state_prediction = A*prev_state + [Ts 0; 0 0]*[ctrl_input_gyro; 0 ];
covariance_prediction = A*covariance_correction_prev*A' + Q;

%-------------------------------
%-------------------------------
%---- Estimate Stage -----------
%-------------------------------
%-------------------------------

    %H matrix
    H = [1 0];

    %Measurement noise from accelerometer angle measurement
    m_var = 0.9;
%     m_var_r = 1;

    R = [m_var^2 ];

    %Measurement Z
    Z = [measurement_angle];

    %Compute Kalman Gain
    Kalman_Gain = covariance_prediction*H'*inv(H*covariance_prediction*H'+R); %2x2 matrix

    %compute state space correction based on measurement
    state_correction = state_prediction + Kalman_Gain*(Z - H*state_prediction); %4x1 vector of states

    %compute covariance correction
    covariance_correction = (eye(2) - Kalman_Gain*H)*covariance_prediction; %2x2 covariance matrix

%     corrected_angle_measure = state_correction(1) - Ts*state_correction(2);
end

== matlab function ardrone_alphaepsilon/Navigation System1/Kalman Filter/Compute Roll Pitch/KF_ROLL/Kalman Tracker ==
  data: prev_state input; covariance_correction_prev input; state_correction output; covariance_correction output; ctrl_input_gyro input; measurement_angle input
function [state_correction, covariance_correction] = fcn(prev_state, covariance_correction_prev, ctrl_input_gyro, measurement_angle)


%-------------------------------
%-------------------------------
%---- Predict Stage ------------
%-------------------------------
%-------------------------------
% pix_value = 5;
Ts = 1/400;
%Process Noise
p_var =0.01;
Q = [p_var^2     0         
      0         p_var^2];

%A matrix
A =  [1   -Ts 
      0   1];

%odutput these values with a unit delay (for algebraic loop), apply initial conditions
state_prediction = A*prev_state + [Ts 0; 0 0]*[ctrl_input_gyro; 0 ];
covariance_prediction = A*covariance_correction_prev*A' + Q;

%-------------------------------
%-------------------------------
%---- Estimate Stage -----------
%-------------------------------
%-------------------------------

    %H matrix
    H = [1 0];

    %Measurement noise from accelerometer angle measurement
    m_var = 0.8;
%     m_var_r = 1;

    R = [m_var^2 ];

    %Measurement Z
    Z = [measurement_angle];

    %Compute Kalman Gain
    Kalman_Gain = covariance_prediction*H'*inv(H*covariance_prediction*H'+R); %2x2 matrix

    %compute state space correction based on measurement
    state_correction = state_prediction + Kalman_Gain*(Z - H*state_prediction); %4x1 vector of states

    %compute covariance correction
    covariance_correction = (eye(2) - Kalman_Gain*H)*covariance_prediction; %2x2 covariance matrix

%     corrected_angle_measure = state_correction(1) - Ts*state_correction(2);
end

== matlab function ardrone_alphaepsilon/Navigation System1/Kalman Filter/Ultrasound  /Kalman Tracker ==
  data: UltraSoundMeasure input; state_correction output; covariance_correction output; covariance_correction_input input; state_correction_input input
function [state_correction, covariance_correction] = fcn(UltraSoundMeasure, covariance_correction_input,state_correction_input)


%-------------------------------
%-------------------------------
%---- Predict Stage ------------
%-------------------------------
%-------------------------------

%our states:
%  [Wx Wy Wz Bx By Bz   ]
%

p_var = 1e-2;
Ts = 1/400;
%Process Noise

Q = [p_var^2     0     
      0         p_var^2 ];

%A matrix
A =  [1   Ts    
      0   1];

%odutput these values with a unit delay (for algebraic loop), apply initial conditions
state_prediction = A*state_correction_input;
covariance_prediction_ = A*covariance_correction_input*A' + Q;

%-------------------------------
%-------------------------------
%---- Estimate Stage -----------
%-------------------------------
%-------------------------------
    %H matrix
    H = [1 0];

    %Measurement noise
    m_var = 1;
%     m_var_r = 1;

    R = [m_var^2];

    %Measurement Z
    Z = UltraSoundMeasure;

    %Compute Kalman Gain
    Kalman_Gain = covariance_prediction_*H'*inv(H*covariance_prediction_*H'+R); %2x2 matrix

    %compute state space correction based on measurement
    state_correction = state_prediction + Kalman_Gain*(Z - H*state_prediction); %2x1 vector of states

    %compute covariance correction
    covariance_correction = (eye(2) - Kalman_Gain*H)*covariance_prediction_; %2x2 covariance matrix

end

== matlab function ardrone_alphaepsilon/Navigation System1/Measurement calibration correction/MATLAB Function ==
  data: Ultrasound_Measure input; UltraSound_Calculation output
function UltraSound_Calculation = removePeak(Ultrasound_Measure)
%#codegen

peakThreshold = 10000;

persistent validHeight
if isempty(validHeight)
    validHeight = 0;
end

if Ultrasound_Measure < peakThreshold
    validHeight = (Ultrasound_Measure - 880) / 26.533;
end

UltraSound_Calculation = validHeight;
